simulink model "CheckBrakeDistance"  (Simulink 7.0)
settings: Solver=ode3  StartTime=0.0  StopTime=inf  RelTol=1e-3
libraries: canoelib x4, simulink x2
settings Model: Creator=visjf  LastModifiedBy=visbma
settings DebuggingCC: MultiTaskCondExecSysMsg=none
settings HardwareCC: TargetHWDeviceType=32-bit Generic
settings RTWCC: SystemTargetFile=cn.tlc  TemplateMakefile=cn_msdll.tmf  Description=Vector CANoe Real-Time Target DLL (Visual C/C++ Project Makefile)  ProcessScript=cn_make_rtw_hook  IncludeERTFirstTime=on
settings STFCustomTargetCC: TargetFcnLib=ansi_tfl_tmw.mat  GenFloatMathFcnCalls=ANSI_C  ModelReferenceCompliant=off  MatFileLogging=on  SystemTargetFile=cn.tlc
settings GRTTargetCC: TargetFcnLib=ansi_tfl_tmw.mat  ModelReferenceCompliant=off  CompOptLevelCompliant=off  ExtModeMexFile=noextcomm  RTWCAPISignals=on  RTWCAPIParams=on
settings CustomProperty: DataType=string  Value=..\..\Exec32

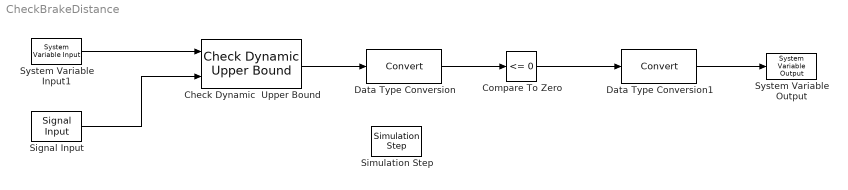
== system CheckBrakeDistance ==
  Check Dynamic  Upper Bound : simulink/Model Verification/Check Dynamic  Upper Bound  Description=sig < max  SystemSampleTime=-1  enabled=on  stopWhenAssertionFail=off  export=on  icon=graphic
  Compare To Zero : simulink/Logic and Bit Operations/Compare To Zero  SystemSampleTime=-1  relop=<=  LogicOutDataTypeMode=uint8  ZeroCross=off
  Data Type Conversion : DataTypeConversion  OutDataType=sfix(16)  OutScaling=2^0
  Data Type Conversion1 : DataTypeConversion  OutDataType=sfix(16)  OutScaling=2^0
  Signal Input : canoelib/CANoe I//O/Signal Input  SystemSampleTime=-1  dbName=""  nodeName=""  msgName=""  sigName=xF  editSampleTime=0  rawValue=off
      settings: AttributesFormatString=%<sigName>
  Simulation Step : canoelib/CANoe I//O/Simulation Step  SystemSampleTime=-1  mode=Synchronized
      settings: AttributesFormatString=%<mode>
  System Variable Input1 : canoelib/CANoe I//O/System Variable Input  SystemSampleTime=-1  nsName=MatlabIO  sysVarName=SetPointBrakeDist  arrayIndex=-1  editSampleTime=0
      settings: AttributesFormatString=%<nsName>::%<sysVarName>
  System Variable Output : canoelib/CANoe I//O/System Variable Output  SystemSampleTime=-1  nsName=MatlabIO  sysVarName=BrakeDistVerdict  arrayIndex=-1
      settings: AttributesFormatString=%<nsName>::%<sysVarName>
  wires:
  System Variable Input1/1 -> Check Dynamic  Upper Bound/1
  Signal Input/1 -> Check Dynamic  Upper Bound/2
  Check Dynamic  Upper Bound/1 -> Data Type Conversion/1
  Data Type Conversion/1 -> Compare To Zero/1
  Compare To Zero/1 -> Data Type Conversion1/1
  Data Type Conversion1/1 -> System Variable Output/1
